simulink model "nn_control"  (R2023a)
settings: Solver=VariableStepAuto  StartTime=0.0  StopTime=400  RelTol=1e-3
values from neighbouring files (symbols this model uses):
  A1 = 0.0154    [parametros.m]    (also in variables.mat)
  A2 = 5e-5    (= 5e-05)    [parametros.m]    (also in variables.mat)
  az = 0.5    [parametros.m]    (also in variables.mat)
  g = 9.8    [parametros.m]    (also in variables.mat)
  H_star = H_max/2    (= 0.31)    [parametros.m]    (also in variables.mat)
  ro = 1000    [parametros.m]    (also in variables.mat)
settings Model: Creator=empg0  LastModifiedBy=empg0

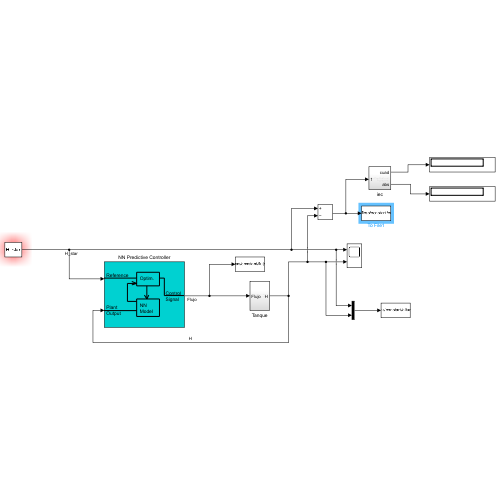
[thumbnail: Simulink's stored preview of the top-level diagram]
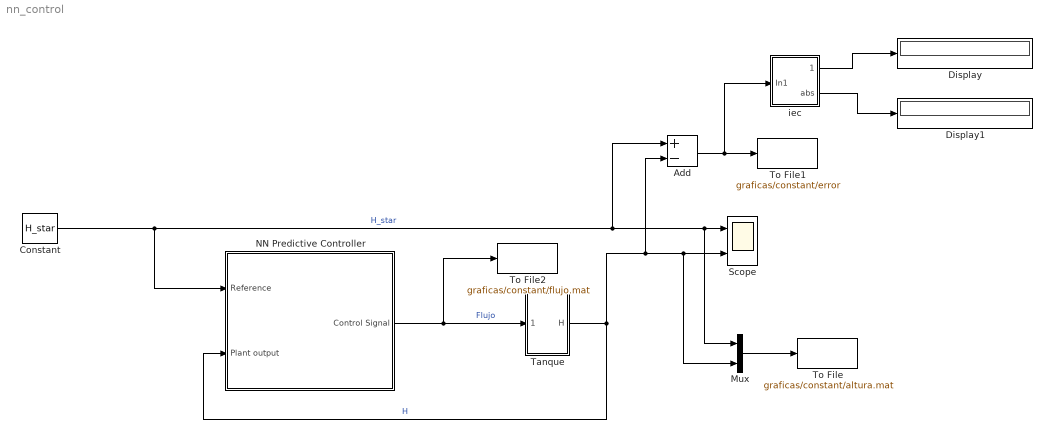
== system nn_control ==
  Add : Sum  Inputs=+-
  Constant : Constant  Value=H_star
  Display : Display
  Display1 : Display
  Mux : Mux  Inputs=2
  NN Predictive Controller : Subsystem  mask(NN Predictive Controller){N2=7, Nu=2, Ts=0.5, rho=0.05, alpha=0.001, csrchfun=csrchbac, maxiter=2, S1=7, Ni=2, Nj=2, sim_file=planta, trainfun=trainlm, Use_validation=1, Use_Testing=0, max_i=0.1, min_i=0, sam_training=8000, epochs=200, minp=0.00083750919477898130849, maxp=0.099220790480832016245, mint=0, maxt=0.099220790480832016245, Normalize=0, IW=[-20.531676995171057598 18.704335179754611573;0.00020386653261894715898 -0.00065105597203892015979;0.11039206030581787121 0.078287285196172784474;-4.2899902912608469663 -2.5279624927180339711;-7.6432027343615454029 11.5285765668885265;-0.017993776662611957878 0.0088727669270464385592;-9.0344400995814524435 3.9540417662274571775], LW1_2=[14.923957143723018959 -17.978284009820111322;-0.71975082637667153751 0.32012412094941411489;0.64966823503412085561 0.085723391515673319496;55.495721009703864013 -51.282194417149113974;-3.6640121805562331225 2.3449172788885150887;-0.52558872900568831543 0.055226005018602114527;-1.7503201452350198863 4.144472061218764658], LW2_1=[-2.1959814678618032602 -3.2437397056361580994 7.2781964126742613175 2.1984051114526992343 1.7353616977917190045 -2.0712307468921604681 2.1983321974786087516], B1=[18.564420214207171256;9.6247423275479970783;-3.5269187756800972622;-67.658376524939384922;-4.4107470426168395861;0.061944283876979457093;-40.321949269656272463], B2=18.964938123059841502, max_i_int=20, min_i_int=5, limit_output=1, max_output=0.62, min_output=0, Use_Previous_Weights=1}
      mask prompts: Ts "Sample time"; rho "rho (typically = 0.03)"; alpha "alpha (typically = 0.001)"; csrchfun "Minimization rutine"; trainfun "Training function"
      mask help: NN Predictive Controller. You first train a neural network model of the plant to be controlled. The controller uses the plant model to predict plant performance over a specified time horizon. An optimization algorithm determines the control signal that optimizes plant performance over this horizon. Double click the NN Predictive Controller block to train the plant model and set the controller parameters.
      mask init:
      | xl = [0   .53   .53     .85   .85  .53  .53  NaN .85  .92 .92];
      | yl = [.95 .95 1.05  1.05   .82  .82  .95  NaN  .95 .95 .65];
      | x2 = [0 .53    NaN .92 1.2 NaN .53 .85 .85 .53 .53 ];
      | y2 = [.39 .39   NaN .65 .65 NaN .59 .59 .29 .29  .59];
      | x3 = [.67 .67 NaN .64 .67 .70 NaN .53 .4   .4   .53 NaN .46 .53 .46];
      | y3 = [.59 .82 NaN .66 .59 .66 NaN .55 .55 .86 .86 NaN  .89 .86 .83];
      | 
      | x1t=.03; y1t=.31;
      | x2t=.03; y2t=.8;
      | x8t=.03;y8t=.21;
      | x3t=.77; y3t=.53;
      | x4t=.77; y4t=.44;
      | x5t=.45; y5t=.76;
      | x6t=.45; y6t=.35;
      | x7t=.45; y7t=.25;
      settings: OpenFcn=nncontrolutil('nnpredict','',gcbh,gcb);
      mask TypeOptions csrchfun: csrchgol | csrchbac | csrchhyb | csrchbre | csrchcha
      mask TypeOptions trainfun: trainbfg | trainbr  | traincgb | traincgf | traincgp | traingd | traingdm | traingda | traingdx | trainlm  | trainoss | trainrp  | trainscg
      mask Display:
      | plot([[xl NaN x2]*.9-.075 ], [[yl  NaN y2]*.9-.1 ]);
      | plot([[x3]*.9-.075 ], [[y3]*.9-.1 ]);
      | text(x1t,y1t,'Plant');
      | text(x8t,y8t,'Output');
      | text(x2t,y2t,'Reference');
      | text(x3t,y3t,'Control');
      | text(x4t,y4t,'Signal');
      | text(x5t,y5t,'Optim.');
      | text(x6t,y6t,'NN');
      | text(x7t,y7t,'Model');
  Scope : Scope  NumInputPorts=2
  Tanque : Subsystem
  To File : ToFile  Filename=graficas/constant/altura.mat  MatrixName=altura  SampleTime=0.5
  To File1 : ToFile  Filename=graficas/constant/error  MatrixName=error  SampleTime=0.5
  To File2 : ToFile  Filename=graficas/constant/flujo.mat  MatrixName=flujo  SampleTime=0.5
  iec : Subsystem
  wires:
  Constant/1 -> NN Predictive Controller/1(Reference), Add/1, Mux/1, Scope/1  "H_star"
  Tanque/1(H) -> Add/2, Mux/2, Scope/2, NN Predictive Controller/2(Plant output)  "H"
  NN Predictive Controller/1(Control Signal) -> To File2/1, Tanque/1(Flujo)  "Flujo"
  Mux/1 -> To File/1
  Add/1 -> iec/1(In1), To File1/1
  iec/1(cuad) -> Display/1
  iec/2(abs) -> Display1/1

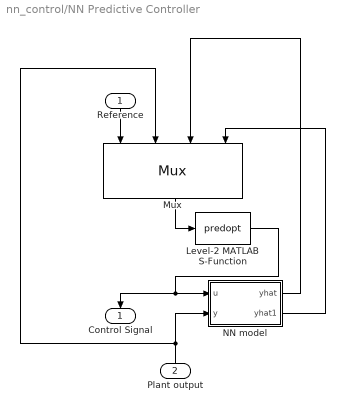
== system nn_control/NN Predictive Controller ==
  Reference : Inport
  Plant output : Inport  Port=2
  Level-2 MATLAB S-Function : M-S-Function  FunctionName=predopt  Parameters=N2,Ts,Nu,maxiter,csrchfun,rho,alpha,S1,IW,LW1_2,LW2_1,B1,B2,Ni,Nj,min_i,max_i,minp,maxp,mint,maxt,Normalize
  Mux : Mux
      settings: DisplayOption=signals
  NN model : Subsystem
  Control Signal : Outport
  wires:
  Mux/1 -> Level-2 MATLAB S-Function/1
  Level-2 MATLAB S-Function/1 -> NN model/1(u), Control Signal/1
  NN model/2(yhat1) -> Mux/4
  NN model/1(yhat) -> Mux/3
  Reference/1 -> Mux/1
  Plant output/1 -> NN model/2(y), Mux/2

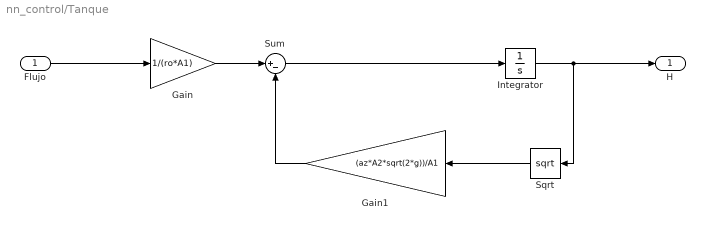
== system nn_control/Tanque ==
  Flujo : Inport
  Gain : Gain  Gain=1/(ro*A1)
  Gain1 : Gain  Gain=(az*A2*sqrt(2*g))/A1
  Integrator : Integrator  LimitOutput=on  UpperSaturationLimit=0.62  LowerSaturationLimit=0
  Sqrt : Sqrt
  Sum : Sum  Inputs=|+-
  H : Outport
  wires:
  Gain/1 -> Sum/1
  Sum/1 -> Integrator/1
  Sqrt/1 -> Gain1/1
  Gain1/1 -> Sum/2
  Integrator/1 -> H/1, Sqrt/1
  Flujo/1 -> Gain/1

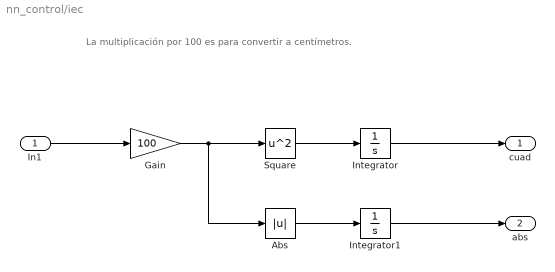
== system nn_control/iec ==
  note: La multiplicación por 100 es para convertir a centímetros.
  In1 : Inport
  Abs : Abs  SaturateOnIntegerOverflow=off
  Gain : Gain  Gain=100
  Integrator : Integrator
  Integrator1 : Integrator
  Square : Math  Operator=square  SignedPower=on  RndMeth=Zero
  cuad : Outport
  abs : Outport  Port=2
  wires:
  Square/1 -> Integrator/1
  Integrator/1 -> cuad/1
  In1/1 -> Gain/1
  Gain/1 -> Abs/1, Square/1
  Abs/1 -> Integrator1/1
  Integrator1/1 -> abs/1

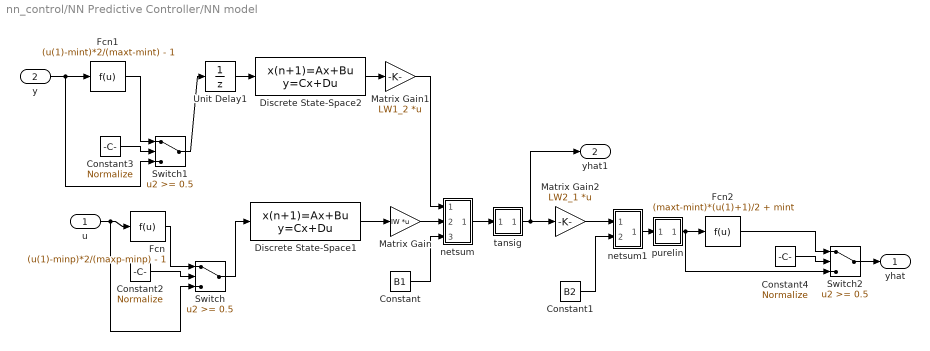
== system nn_control/NN Predictive Controller/NN model ==
  u : Inport
  y : Inport  Port=2
  Constant : Constant  Value=B1
  Constant1 : Constant  Value=B2
  Constant2 : Constant  Value=Normalize
  Constant3 : Constant  Value=Normalize
  Constant4 : Constant  Value=Normalize
  Discrete State-Space1 : DiscreteStateSpace  A=[0 zeros(1,Ni-2);eye(Ni-2,Ni-1)]  B=[zeros(double(Ni==1));eye(Ni-1,1)]  C=[0 zeros(1,Ni-2);eye(Ni-1,Ni-1)]  D=eye(Ni,1)  SampleTime=Ts
  Discrete State-Space2 : DiscreteStateSpace  A=[0 zeros(1,Nj-2);eye(Nj-2,Nj-1)]  B=[zeros(double(Nj==1));eye(Nj-1,1)]  C=[0 zeros(1,Nj-2);eye(Nj-1,Nj-1)]  D=eye(Nj,1)  SampleTime=Ts
  Fcn : Fcn  Expr=(u(1)-minp)*2/(maxp-minp) - 1
  Fcn1 : Fcn  Expr=(u(1)-mint)*2/(maxt-mint) - 1
  Fcn2 : Fcn  Expr=(maxt-mint)*(u(1)+1)/2 + mint
  Matrix Gain : Gain  Gain=IW  Multiplication=Matrix(K*u)  SaturateOnIntegerOverflow=on  OutDataTypeStr=Inherit: Same as input  ParamDataTypeStr=Inherit: Same as input
  Matrix Gain1 : Gain  Gain=LW1_2  Multiplication=Matrix(K*u)  SaturateOnIntegerOverflow=on  OutDataTypeStr=Inherit: Same as input  ParamDataTypeStr=Inherit: Same as input
  Matrix Gain2 : Gain  Gain=LW2_1  Multiplication=Matrix(K*u)  SaturateOnIntegerOverflow=on  OutDataTypeStr=Inherit: Same as input  ParamDataTypeStr=Inherit: Same as input
  Switch : Switch  Threshold=0.5  ZeroCross=off
  Switch1 : Switch  Threshold=0.5  ZeroCross=off
  Switch2 : Switch  Threshold=0.5  ZeroCross=off
  Unit Delay1 : UnitDelay  SampleTime=Ts  HasFrameUpgradeWarning=on
  netsum : Subsystem
      mask Display: disp('+')
  netsum1 : Subsystem
      mask Display: disp('+')
  purelin : Subsystem
      mask Display: plot([-1 1],[0 0],[-1 1],[-1 1])
  tansig : Subsystem
      mask Display: plot([-1 1],[0 0],[-1 -.9 -.8 -.7 -.6 -.5 -.4 -.3 -.2 -.1 0 .1 .2 .3 .4 .5 .6 .7 .8 .9 1],2./(1+exp(-8*[-1 -.9 -.8 -.7 -.6 -.5 -.4 -.3 -.2 -.1 0 .1 .2 .3 .4 .5 .6 .7 .8 .9 1]))-1)
  yhat : Outport
  yhat1 : Outport  Port=2
  wires:
  netsum1/1(Out1) -> purelin/1(n)
  Constant1/1 -> netsum1/2(In2)
  Matrix Gain2/1 -> netsum1/1(In1)
  netsum/1(Out1) -> tansig/1(n)
  Constant/1 -> netsum/3(In3)
  Matrix Gain1/1 -> netsum/1(In1)
  Matrix Gain/1 -> netsum/2(In2)
  tansig/1(a) -> Matrix Gain2/1, yhat1/1
  Discrete State-Space1/1 -> Matrix Gain/1
  Fcn/1 -> Switch/1
  Switch/1 -> Discrete State-Space1/1
  u/1 -> Fcn/1, Switch/3
  Constant2/1 -> Switch/2
  Discrete State-Space2/1 -> Matrix Gain1/1
  Unit Delay1/1 -> Discrete State-Space2/1
  Constant3/1 -> Switch1/2
  Switch1/1 -> Unit Delay1/1
  Fcn1/1 -> Switch1/1
  y/1 -> Fcn1/1, Switch1/3
  Constant4/1 -> Switch2/2
  Switch2/1 -> yhat/1
  Fcn2/1 -> Switch2/1
  purelin/1(a) -> Fcn2/1, Switch2/3

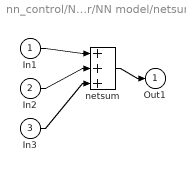
== system nn_control/NN Predictive Controller/NN model/netsum ==
  In1 : Inport
  In2 : Inport  Port=2
  In3 : Inport  Port=3
  netsum : Sum  Inputs=3  InputSameDT=on  SaturateOnIntegerOverflow=on  OutDataTypeStr=Inherit: Same as first input
  Out1 : Outport
  wires:
  In1/1 -> netsum/1
  In2/1 -> netsum/2
  In3/1 -> netsum/3
  netsum/1 -> Out1/1

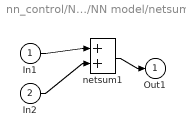
== system nn_control/NN Predictive Controller/NN model/netsum1 ==
  In1 : Inport
  In2 : Inport  Port=2
  netsum1 : Sum  Inputs=2  InputSameDT=on  SaturateOnIntegerOverflow=on  OutDataTypeStr=Inherit: Same as first input
  Out1 : Outport
  wires:
  In1/1 -> netsum1/1
  In2/1 -> netsum1/2
  netsum1/1 -> Out1/1

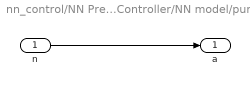
== system nn_control/NN Predictive Controller/NN model/purelin ==
  n : Inport
  a : Outport
  wires:
  n/1 -> a/1

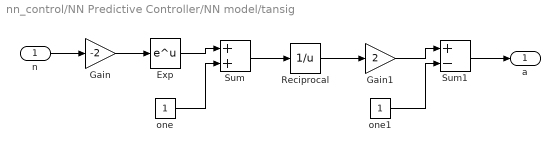
== system nn_control/NN Predictive Controller/NN model/tansig ==
  n : Inport
  Exp : Math  SignedPower=on
  Gain : Gain  Gain=-2  SaturateOnIntegerOverflow=on  OutDataTypeStr=Inherit: Same as input  ParamDataTypeStr=Inherit: Same as input
  Gain1 : Gain  Gain=2  SaturateOnIntegerOverflow=on  OutDataTypeStr=Inherit: Same as input  ParamDataTypeStr=Inherit: Same as input
  Reciprocal : Math  Operator=reciprocal  SignedPower=on
  Sum : Sum  InputSameDT=on  SaturateOnIntegerOverflow=on  OutDataTypeStr=Inherit: Same as first input
  Sum1 : Sum  Inputs=+-  InputSameDT=on  SaturateOnIntegerOverflow=on  OutDataTypeStr=Inherit: Same as first input
  one : Constant
  one1 : Constant
  a : Outport
  wires:
  n/1 -> Gain/1
  Gain/1 -> Exp/1
  Exp/1 -> Sum/1
  one/1 -> Sum/2
  Sum/1 -> Reciprocal/1
  Reciprocal/1 -> Gain1/1
  Gain1/1 -> Sum1/1
  one1/1 -> Sum1/2
  Sum1/1 -> a/1
